simulink model "FXP_AFMss_obshas_uk"  (R2018b)
settings: Solver=ode4  StartTime=0.0  StopTime=trun  FixedStep=Ts  RelTol=1e-5  EnableMultiTasking=on
PreLoadFcn:
  | VSS_CONTROL_MODE=1;
  | VSS_LINEAR_CONTROL=Simulink.Variant('VSS_CONTROL_MODE==1');
  | VSS_MPC_CONTROL=Simulink.Variant('VSS_CONTROL_MODE == 2');
  | 
  | 
  | VSS_STATE_DIRECT=Simulink.Variant('VSS_STATE_MODE==1');
  | VSS_STATE_OBS=Simulink.Variant('VSS_STATE_MODE==2');
  | VSS_STATE_DIST_OBS=Simulink.Variant('VSS_STATE_MODE==3');
  | VSS_STATE_MODE=1;
undefined symbols (not defined in the file): C_ydist, d, dp, Ident_obs, K_lqr, r, rp, sim_obj, sim_struct, Ts, w, wp, ws, wsp
libraries: cstblocks x4
settings Model: MinMaxOverflowLogging=MinMaxAndOverflow  FPTRunName=NoOverride  Creator=arnold  LastModifiedBy=arnold
settings DataIOCC: SaveFormat=Array  SaveOutput=off  SaveState=on  InspectSignalLogs=on  TimeSaveName=tout_ptos
settings OptimizationCC: LifeSpan=inf
settings DebuggingCC: SolverPrmCheckMsg=warning  LibraryContextMissingDiagnostic=none  SFUnexpectedBacktrackingDiag=warning  SFNoUnconditionalDefaultTransitionDiag=warning  SFExecutionAtInitializationDiag=none
settings HardwareCC: ProdBitPerPointer=32  ProdBitPerSizeT=32  ProdBitPerPtrDiffT=32  ProdLargestAtomicFloat=None  ProdIntDivRoundTo=Undefined  ProdEndianess=Unspecified  ProdWordSize=32  ProdHWDeviceType=32-bit Generic
settings ModelReferenceCC: PropagateSignalLabelsOutOfModel=off
settings SFSimCC: SimUseLocalCustomCode=off
settings RTWCC: RTWUseLocalCustomCode=off
settings CodeAppCC: StateflowObjectComments=on
settings GRTTargetCC: TargetLangStandard=C89/C90 (ANSI)  GeneratePreprocessorConditionals=Disable all
settings ConfigComp: CovMetricSettings=dw  CovHtmlReporting=on  CovSaveCumulativeToWorkspaceVar=on  CovSaveSingleToWorkspaceVar=on  CovExternalEMLEnable=off  CovSFcnEnable=off

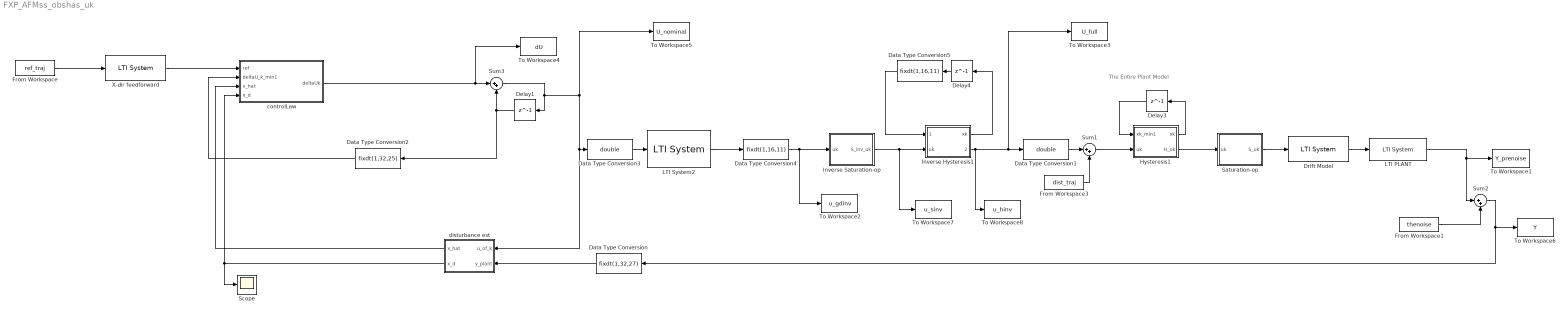
== system FXP_AFMss_obshas_uk ==
  note: The Entire Plant Model
  Data Type Conversion : DataTypeConversion  OutDataTypeStr=fixdt(1,32,27)
  Data Type Conversion1 : DataTypeConversion  OutDataTypeStr=double  LockScale=on
  Data Type Conversion2 : DataTypeConversion  OutDataTypeStr=fixdt(1,32,25)
  Data Type Conversion3 : DataTypeConversion  OutDataTypeStr=double  LockScale=on
  Data Type Conversion4 : DataTypeConversion  OutDataTypeStr=fixdt(1,16,11)  LockScale=on
  Data Type Conversion5 : DataTypeConversion  OutDataTypeStr=fixdt(1,16,11)
  Delay1 : Delay  DelayLength=1  InitialCondition=0  SampleTime=Ts
  Delay3 : Delay  DelayLength=1  InitialCondition=zeros(length(r), 1)
  Delay4 : Delay  DelayLength=1  InitialCondition=fi(zeros(length(rp), 1), 1, 16, 11)
  Drift Model : cstblocks/LTI System  sys=sim_obj.gdrift  IC=x0_full
  From Workspace : FromWorkspace  VariableName=ref_traj  SampleTime=Ts
  From Workspace1 : FromWorkspace  VariableName=thenoise  SampleTime=Ts
  From Workspace3 : FromWorkspace  VariableName=dist_traj  SampleTime=Ts
  Hysteresis1 : MATLAB Function  TreatAsAtomicUnit=on
  Inverse Hysteresis1 : MATLAB Function  TreatAsAtomicUnit=on
  Inverse Saturation-op : MATLAB Function  TreatAsAtomicUnit=on
  LTI PLANT : cstblocks/LTI System  sys=PLANT  IC=[]
  LTI System2 : cstblocks/LTI System  sys=sim_obj.gdrift_inv  IC=[]
  Saturation-op : MATLAB Function  TreatAsAtomicUnit=on
  Scope : Scope
  Sum1 : Sum  Inputs=|++
  Sum2 : Sum  Inputs=|++
  Sum3 : Sum  Inputs=|++  OutDataTypeStr=fixdt(1,32,27)
  To Workspace1 : ToWorkspace  VariableName=Y_prenoise  SaveFormat=Timeseries  SampleTime=-1
      settings: Save2DSignal=2-D array (concatenate along first dimension)
  To Workspace2 : ToWorkspace  VariableName=u_gdinv  SaveFormat=Timeseries  SampleTime=-1
      settings: Save2DSignal=2-D array (concatenate along first dimension)
  To Workspace3 : ToWorkspace  VariableName=U_full  SaveFormat=Timeseries  SampleTime=-1
      settings: Save2DSignal=2-D array (concatenate along first dimension)
  To Workspace4 : ToWorkspace  VariableName=dU  SaveFormat=Timeseries  SampleTime=-1
      settings: Save2DSignal=2-D array (concatenate along first dimension)
  To Workspace5 : ToWorkspace  VariableName=U_nominal  SaveFormat=Timeseries  SampleTime=-1
      settings: Save2DSignal=2-D array (concatenate along first dimension)
  To Workspace6 : ToWorkspace  VariableName=Y  SaveFormat=Timeseries  SampleTime=-1
      settings: Save2DSignal=2-D array (concatenate along first dimension)
  To Workspace7 : ToWorkspace  VariableName=u_sinv  SaveFormat=Timeseries  SampleTime=-1
      settings: Save2DSignal=2-D array (concatenate along first dimension)
  To Workspace8 : ToWorkspace  VariableName=u_hinv  SaveFormat=Timeseries  SampleTime=-1
      settings: Save2DSignal=2-D array (concatenate along first dimension)
  X-dir feedforward : cstblocks/LTI System  sys=sim_obj.Dx_ff  IC=0
  controlLaw : Subsystem
  disturbance est : Subsystem  VariantControl=VSS_STATE_DIST_OBS
  wires:
  Sum2/1 -> Data Type Conversion/1, To Workspace6/1
  Delay1/1 -> Data Type Conversion2/1, Sum3/2
  disturbance est/2(x_d) -> Scope/1, controlLaw/4(x_d)
  Data Type Conversion/1 -> disturbance est/2(y_plant)
  controlLaw/1(deltaUk) -> To Workspace4/1, Sum3/1
  disturbance est/1(x_hat) -> controlLaw/3(x_hat)
  Data Type Conversion2/1 -> controlLaw/2(deltaU_k_min1)
  Drift Model/1 -> LTI PLANT/1
  LTI System2/1 -> Data Type Conversion4/1
  Hysteresis1/1(xk) -> Delay3/1
  Delay3/1 -> Hysteresis1/1(xk_min1)
  Hysteresis1/2(H_uk) -> Saturation-op/1(uk)
  Inverse Hysteresis1/1(xk) -> Delay4/1
  Data Type Conversion5/1 -> Inverse Hysteresis1/1(xk_min1)
  Data Type Conversion1/1 -> Sum1/1
  Sum3/1 -> To Workspace5/1, Data Type Conversion3/1, disturbance est/1(u_of_k), Delay1/1
  Data Type Conversion3/1 -> LTI System2/1
  Inverse Hysteresis1/2(H_inv_uk) -> To Workspace8/1, To Workspace3/1, Data Type Conversion1/1
  Data Type Conversion4/1 -> To Workspace2/1, Inverse Saturation-op/1(uk)
  Delay4/1 -> Data Type Conversion5/1
  Inverse Saturation-op/1(S_inv_uk) -> To Workspace7/1, Inverse Hysteresis1/2(uk)
  Saturation-op/1(S_uk) -> Drift Model/1
  Sum1/1 -> Hysteresis1/2(uk)
  From Workspace3/1 -> Sum1/2
  LTI PLANT/1 -> Sum2/1, To Workspace1/1
  From Workspace1/1 -> Sum2/2
  From Workspace/1 -> X-dir feedforward/1
  X-dir feedforward/1 -> controlLaw/1(ref)

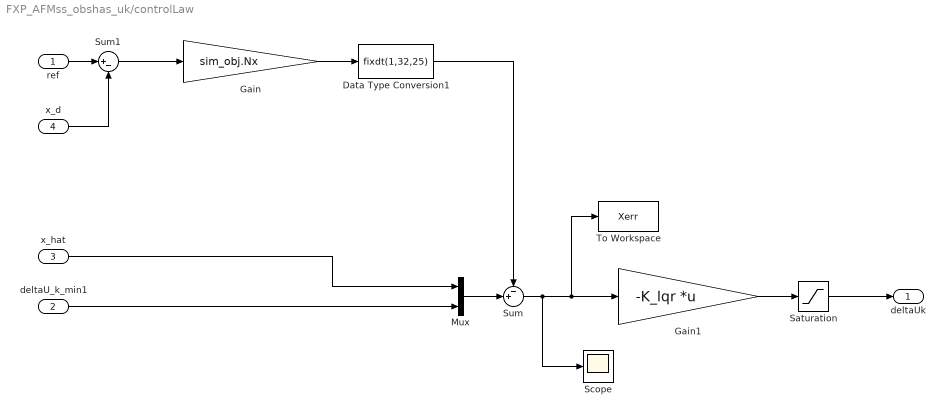
== system FXP_AFMss_obshas_uk/controlLaw ==
  ref : Inport
  deltaU_k_min1 : Inport  Port=2
  x_hat : Inport  Port=3
  x_d : Inport  Port=4
  Data Type Conversion1 : DataTypeConversion  OutDataTypeStr=fixdt(1,32,25)
  Gain : Gain  Gain=sim_obj.Nx  OutDataTypeStr=fixdt(1,sim_obj.nw, sim_obj.nf)
  Gain1 : Gain  Gain=-K_lqr  Multiplication=Matrix(K*u)  OutDataTypeStr=fixdt(1,nw,nf)
  Mux : Mux  Inputs=2
  Saturation : Saturate  UpperLimit=sim_obj.du_max  LowerLimit=-sim_obj.du_max
  Scope : Scope
  Sum : Sum  Inputs=-+|  OutDataTypeStr=fixdt(1,sim_obj.nw, sim_obj.nf)
  Sum1 : Sum  Inputs=|+-
  To Workspace : ToWorkspace  VariableName=Xerr  SaveFormat=Timeseries  SampleTime=-1
  deltaUk : Outport
  wires:
  Saturation/1 -> deltaUk/1
  Gain1/1 -> Saturation/1
  ref/1 -> Sum1/1
  Sum/1 -> Scope/1, Gain1/1, To Workspace/1
  x_hat/1 -> Mux/1
  deltaU_k_min1/1 -> Mux/2
  Mux/1 -> Sum/2
  Gain/1 -> Data Type Conversion1/1
  Sum1/1 -> Gain/1
  x_d/1 -> Sum1/2
  Data Type Conversion1/1 -> Sum/1

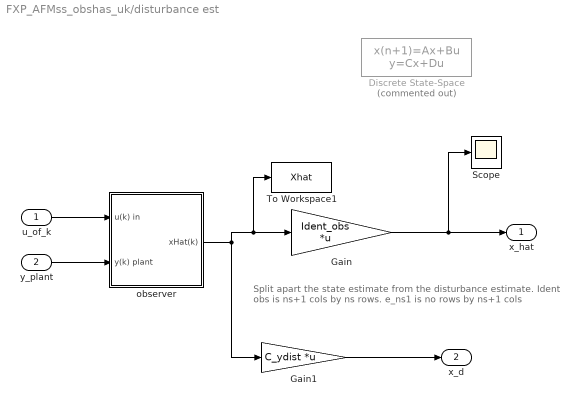
== system FXP_AFMss_obshas_uk/disturbance est ==
  note: Split apart the state estimate from the disturbance estimate.
      | Ident obs is ns+1 cols by ns rows. e_ns1 is no rows by ns+1 cols
  u_of_k : Inport  OutDataTypeStr=fixdt(1,32,27)
  y_plant : Inport  Port=2  OutDataTypeStr=fixdt(1,32,27)
  Discrete State-Space : DiscreteStateSpace  Commented=on  A=sim_struct.sys_obs.a  B=[sim_struct.sys_obs.b, sim_struct.L]  C=eye(length(sim_struct.sys_obs.b))  D=zeros(length(sim_struct.sys_obs.b), 2)  InitialCondition=sim_struct.x0_obs  SampleTime=Ts
  Gain : Gain  Gain=Ident_obs  Multiplication=Matrix(K*u)  OutDataTypeStr=fixdt(1,32,25)
  Gain1 : Gain  Gain=C_ydist  Multiplication=Matrix(K*u)  OutDataTypeStr=fixdt(1,32,27)  LockScale=on
  Scope : Scope
  To Workspace1 : ToWorkspace  VariableName=Xhat  SaveFormat=Timeseries  SampleTime=-1
      settings: Save2DSignal=2-D array (concatenate along first dimension)
  observer : Subsystem
  x_hat : Outport
  x_d : Outport  Port=2
  wires:
  u_of_k/1 -> observer/1(u(k) in)
  observer/1(xHat(k)) -> To Workspace1/1, Gain/1, Gain1/1
  y_plant/1 -> observer/2(y(k) plant)
  Gain/1 -> Scope/1, x_hat/1
  Gain1/1 -> x_d/1

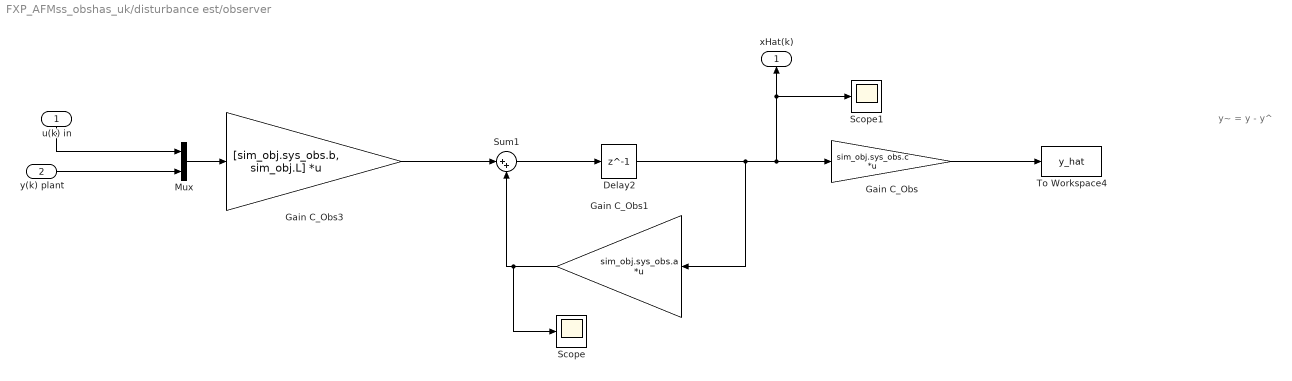
== system FXP_AFMss_obshas_uk/disturbance est/observer ==
  note: y~ = y - y^
  u(k) in : Inport  OutDataTypeStr=fixdt(1,32,27)
  y(k) plant : Inport  Port=2  OutDataTypeStr=fixdt(1,32,27)
  Delay2 : Delay  DelayLength=1  InitialCondition=sim_obj.x0_obs
  Gain C_Obs : Gain  Gain=sim_obj.sys_obs.c  Multiplication=Matrix(K*u)  OutDataTypeStr=fixdt(1,32,27)
  Gain C_Obs1 : Gain  Gain=sim_obj.sys_obs.a  Multiplication=Matrix(K*u)
  Gain C_Obs3 : Gain  Gain=[sim_obj.sys_obs.b, sim_obj.L]  Multiplication=Matrix(K*u)  OutDataTypeStr=fixdt(1,32,25)
  Mux : Mux  Inputs=2
  Scope : Scope
  Scope1 : Scope
  Sum1 : Sum  Inputs=|++  OutDataTypeStr=fixdt(1,32,25)
  To Workspace4 : ToWorkspace  VariableName=y_hat  SaveFormat=Timeseries  SampleTime=-1
      settings: Save2DSignal=2-D array (concatenate along first dimension)
  xHat(k) : Outport
  wires:
  Sum1/1 -> Delay2/1
  Gain C_Obs1/1 -> Scope/1, Sum1/2
  Mux/1 -> Gain C_Obs3/1
  Gain C_Obs/1 -> To Workspace4/1
  Delay2/1 -> Scope1/1, xHat(k)/1, Gain C_Obs/1, Gain C_Obs1/1
  Gain C_Obs3/1 -> Sum1/1
  u(k) in/1 -> Mux/1
  y(k) plant/1 -> Mux/2

== matlab function FXP_AFMss_obshas_uk/Inverse Saturation-op ==
  data: uk input; S_inv_uk output fixdt(1,16,11); wsp parameter; dp parameter fixdt(1,16,11)
function S_inv_uk  = fcn(uk, wsp, dp)
  % Implement simple Saturation model.
%   keyboard

  if length(dp) > 1
    Sd_vec = 0*dp(:);
    for i=1:length(dp)
      if dp(i) == 0
        Sd_vec(i) = uk;
      elseif dp(i) > 0
        Sd_vec(i) = max(uk - dp(i), 0);
      else
        Sd_vec(i) = min(uk - dp(i), 0);
      end
    end
    S_inv_uk = wsp(:)'*Sd_vec;
  else
   S_inv_uk = uk;
  end
  S_inv_uk = fi(S_inv_uk, 1, 16, 11);
end

== matlab function FXP_AFMss_obshas_uk/Hysteresis1 ==
  data: xk output; xk_min1 input; uk input; H_uk output; r parameter; w parameter
function [xk, H_uk] = fcn(xk_min1, uk, r, w)
  % Implement simple IP hysteresis model.
  if length(r) > 1
    xk = r(:)*0;
    for j = 1:length(r)
      xk(j) = max(uk - r(j), min(uk+r(j), xk_min1(j)));
    end
    
    H_uk = w'*xk(:);
  else
    xk = xk_min1;
    H_uk = uk;
  end
end

== matlab function FXP_AFMss_obshas_uk/Inverse Hysteresis1 ==
  data: xk output; xk_min1 input fixdt(1,16,11); uk input; H_inv_uk output; rp parameter; wp parameter
function [xk, H_inv_uk] = fcn(xk_min1, uk, rp, wp)
  % Implement simple IP hysteresis model.
%   keyboard
  if length(rp) > 1
    xk = rp(:)*fi(0, 1, 16, 11);
    for j = 1:length(rp)
      xk(j) = max(uk - rp(j), min(uk+rp(j), xk_min1(j)));
    end
    
    H_inv_uk = wp'*xk(:);
  else
    xk = xk_min1;
    H_inv_uk = uk;
  end
end

== matlab function FXP_AFMss_obshas_uk/Saturation-op ==
  data: uk input; S_uk output; ws parameter; d parameter
function S_uk  = fcn(uk, ws, d)
  % Implement simple Saturation model.
%   keyboard
  if length(d) > 1
    Sd_vec = 0*d(:);
    for i=1:length(d)
      if d(i) == 0
        Sd_vec(i) = uk;
      elseif d(i) > 0
        Sd_vec(i) = max(uk - d(i), 0);
      else
        Sd_vec(i) = min(uk - d(i), 0);
      end
    end
    S_uk = ws(:)'*Sd_vec;
  else
   S_uk = uk;
  end
end
